simulink model "modle"  (R2023a)
settings: Solver=VariableStepAuto  StartTime=0.0  StopTime=10  RelTol=1e-3
model workspace (MAT data in the model file):
  a = 0.05
(part 1 of 2)
settings Model: Creator=shenwei  LastModifiedBy=shenwei

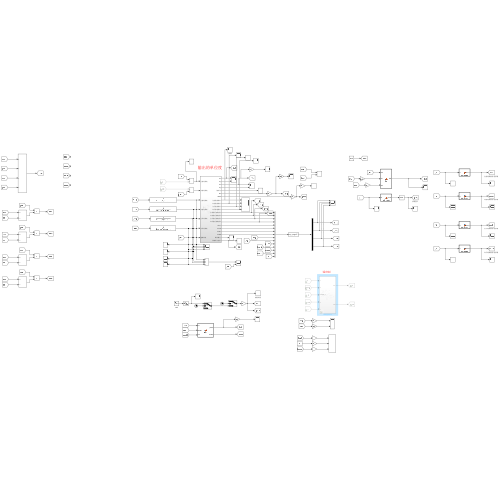
[thumbnail: Simulink's stored preview of the top-level diagram]
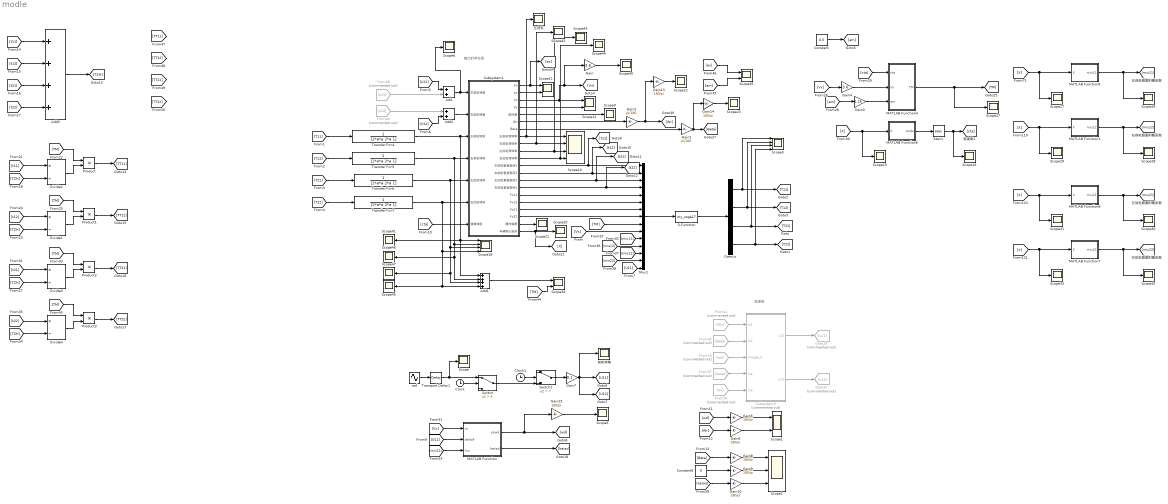
== system modle ==
  note: 输出的单位度
  note: 弧度制
  Add : Sum
  Add1 : Sum  Inputs=++++
  Add2 : Sum
  Add3 : Sum  Inputs=++++
  Atan1 : Trigonometry  Operator=atan
  Clock : Clock
  Clock1 : Clock
  Constant : Constant  Value=0.5
  Constant6 : Constant  Value=0
  Demux : Demux
  Divide{1..4} (4 alike) : Product  Inputs=*/
  From10 : From  Commented=on  GotoTag=wd
  From39 : From  Commented=on  GotoTag=u11
  From40 : From  Commented=on  GotoTag=u12
  From41 : From  Commented=on  GotoTag=Wr
  From42 : From  Commented=on  GotoTag=Beta
  From56 : From  Commented=on  GotoTag=Vx
  From57 : From  Commented=on  GotoTag=betad
  Gain : Gain  Gain=3.6
  Gain1 : Gain  Gain=pi/180
  Gain{5..6,8..10,13..15} (8 alike) : Gain  Gain=180/pi
  Gain2 : Gain  Gain=pi/180
  Gain3 : Gain  Gain=1.28
  Gain4 : Gain  Gain=3.6
  Gain7 : Gain  Gain=0.1
  Goto29 : Goto  Commented=on  GotoTag=u11
  Goto31 : Goto  Commented=on  GotoTag=u12
  MATLAB Function : MATLAB Function  TreatAsAtomicUnit=on
  MATLAB Function1 : MATLAB Function  TreatAsAtomicUnit=on
  MATLAB Function4 : MATLAB Function  TreatAsAtomicUnit=on
  MATLAB Function6 : MATLAB Function  TreatAsAtomicUnit=on
  MATLAB Function7 : MATLAB Function  TreatAsAtomicUnit=on
  MATLAB Function8 : MATLAB Function  TreatAsAtomicUnit=on
  MATLAB Function9 : MATLAB Function  TreatAsAtomicUnit=on
  Mux1 : Mux  Inputs=15
  Product{,1..3} (4 alike) : Product
  S-Function : S-Function  FunctionName=my_nsga17  SFunctionDeploymentMode=off  EnableBusSupport=off
  Scope{,5..6,9,16..17,19..23,26..33,40..47} (27 alike) : Scope
  Scope{1,11..12,34..35} (5 alike) : Scope  NumInputPorts=2
  Scope10 : Scope  NumInputPorts=4
  Scope18 : Scope  NumInputPorts=4
  Scope2 : Scope  NumInputPorts=3
  Scope3 : Scope  NumInputPorts=4
  Subsystem1 : Subsystem
  Subsystem3 : Subsystem  Commented=on
  Switch : Switch  Criteria=u2 > Threshold  Threshold=3  SaturateOnIntegerOverflow=off  InputSameDT=off
  Switch1 : Switch  Criteria=u2 > Threshold  Threshold=7  SaturateOnIntegerOverflow=off  InputSameDT=off
  Transfer Fcn{4..7} (4 alike) : TransferFcn  Denominator=[2*a*a 2*a 1]
  Transport Delay1 : TransportDelay  DelayTime=3
  rad : Sin  Amplitude=pi/4  Frequency=pi/2  SampleTime=0
  前轮转角 : Scope
  左前轮 : Scope
  wires:
  Subsystem1/12(左前轮垂直载荷1) -> [t11], Mux1/1
  Subsystem1/19(Fx22) -> Mux1/8
  Subsystem1/18(Fx21) -> Mux1/7
  Subsystem1/17(Fx12) -> Mux1/6
  Subsystem1/16(Fx11) -> Mux1/5
  Subsystem1/15(右后轮垂直载荷1) -> [t22], Mux1/4
  Subsystem1/14(左后轮垂直载荷1) -> Mux1/3, [t21]
  Subsystem1/13(右前轮垂直载荷1) -> Mux1/2, [t12]
  [TM] -> Mux1/9
  Demux/1 -> Scope3/1, [T11]
  Demux/2 -> Scope3/2, [T12]
  Demux/4 -> Scope3/4, [T22]
  Demux/3 -> Scope3/3, [T21]
  [Vx] -> Mux1/10
  Mux1/1 -> S-Function/1
  S-Function/1 -> Demux/1
  Subsystem1/11(右后轮滑转率) -> Scope44/1, Scope10/4
  Subsystem1/10(左后轮滑转率) -> Scope10/3, Scope43/1
  Subsystem1/9(右前轮滑转率) -> Scope42/1, Scope10/2
  Subsystem1/8(左前轮滑转率) -> Scope10/1, 左前轮/1
  Gain4/1 -> MATLAB Function4/2(Vx)
  MATLAB Function4/1(TM) -> Scope17/1, [TM]
  [cta] -> MATLAB Function4/1(cta)
  [am] -> Gain3/1
  MATLAB Function6/1(podu) -> Atan1/1
  [Vx] -> Gain4/1
  Atan1/1 -> Scope16/1, [cta]
  [cta] -> Subsystem1/7(道路坡度)
  Subsystem1/2(ay) -> Scope11/2
  Subsystem1/4(Vy) -> Scope12/2
  Subsystem1/3(Vx) -> Gain/1, [Vx], Scope12/1
  [X] -> Scope19/1, MATLAB Function6/1(X)
  Gain3/1 -> MATLAB Function4/3(am)
  Transfer Fcn4/1 -> Scope41/1, Scope18/1, Add1/1, Subsystem1/3(左前轮转矩)
  Transfer Fcn7/1 -> Scope45/1, Add1/4, Scope18/4, Subsystem1/6(右后轮转矩)
  Transfer Fcn6/1 -> Scope18/3, Scope47/1, Add1/3, Subsystem1/5(左后轮转矩)
  Transfer Fcn5/1 -> Scope18/2, Scope46/1, Add1/2, Subsystem1/4(右前轮转矩)
  Subsystem1/1(ax) -> [ax], Scope11/1
  MATLAB Function7/1(miu22) -> Scope32/1, [miu22]
  [X] -> Scope31/1, MATLAB Function8/1(X)
  [X] -> Scope33/1, MATLAB Function7/1(X)
  MATLAB Function8/1(miu21) -> Scope30/1, [miu21]
  MATLAB Function9/1(miu11) -> Scope26/1, [miu11]
  [X] -> Scope29/1, MATLAB Function1/1(X)
  [X] -> Scope27/1, MATLAB Function9/1(X)
  MATLAB Function1/1(miu12) -> Scope28/1, [miu12]
  Subsystem1/21(车辆质心坐标) -> Scope20/1, [X]
  [miu11] -> Mux1/11
  [miu12] -> Mux1/12
  [miu21] -> Mux1/13
  [miu22] -> Mux1/14
  Subsystem1/20(横向偏差) -> Scope21/1
  Subsystem1/7(Beta) -> Gain1/1
  Subsystem1/5(航向角) -> Scope9/1
  Subsystem1/6(Wr) -> Gain2/1
  From57/1 -> Subsystem3/4(In4)
  From42/1 -> Subsystem3/2(In2)
  From41/1 -> Subsystem3/1(In1)
  Add1/1 -> Scope34/1
  [TM] -> Scope34/2
  [ax] -> Scope35/1
  [am] -> Scope35/2
  Gain/1 -> Scope40/1
  Constant/1 -> [am]
  Clock1/1 -> Switch1/2
  Switch1/1 -> Gain7/1
  Switch/1 -> Switch1/3
  Transport Delay1/1 -> Switch/1, Scope/1
  Clock/1 -> Switch/2
  rad/1 -> Transport Delay1/1
  [U11] -> Add/1
  From39/1 -> Add/2
  [U12] -> Add2/2
  From40/1 -> Add2/1
  Add/1 -> Scope6/1, Subsystem1/1(左前轮转角)
  Add2/1 -> Subsystem1/2(右前轮转角)
  [U11] -> Mux1/15
  [wd] -> Gain5/1
  [Beta] -> Gain8/1
  Constant6/1 -> Gain9/1
  From10/1 -> Subsystem3/3(omega_d)
  [Wr] -> Gain6/1
  Subsystem3/1(u11) -> Goto29/1
  Subsystem3/2(u12) -> Goto31/1
  [t22] -> Add3/4
  [t11] -> Add3/1
  [t12] -> Add3/2
  [t21] -> Add3/3
  Add3/1 -> [TZH]
  [TZH] -> Divide2/2
  [t11] -> Divide2/1
  Divide2/1 -> Product/2
  [TM] -> Product/1
  Product/1 -> [TT11]
  Divide1/1 -> Product1/2
  [t12] -> Divide1/1
  [TZH] -> Divide1/2
  Product1/1 -> [TT12]
  [TM] -> Product1/1
  Divide3/1 -> Product2/2
  [t21] -> Divide3/1
  [TZH] -> Divide3/2
  Product2/1 -> [TT21]
  [TM] -> Product2/1
  Divide4/1 -> Product3/2
  [t22] -> Divide4/1
  [TZH] -> Divide4/2
  Product3/1 -> [TT22]
  [TM] -> Product3/1
  [Vx] -> MATLAB Function/1(vx)
  [miu11] -> MATLAB Function/3(mu)
  Gain7/1 -> [U12], 前轮转角/1, [U11]
  MATLAB Function/2(betad) -> [betad]
  Gain2/1 -> Gain13/1, [Wr]
  Gain1/1 -> Gain14/1, [Beta]
  Gain5/1 -> Scope1/1
  Gain9/1 -> Scope2/2
  Gain8/1 -> Scope2/1
  Gain6/1 -> Scope1/2
  [betad] -> Gain10/1
  Gain10/1 -> Scope2/3
  MATLAB Function/1(yawd) -> Gain15/1, [wd]
  [U11] -> MATLAB Function/2(deltaf)
  Gain13/1 -> Scope22/1
  Gain14/1 -> Scope23/1
  From56/1 -> Subsystem3/5(In3)
  Gain15/1 -> Scope5/1
  [T11] -> Transfer Fcn4/1
  [T12] -> Transfer Fcn5/1
  [T21] -> Transfer Fcn6/1
  [T22] -> Transfer Fcn7/1

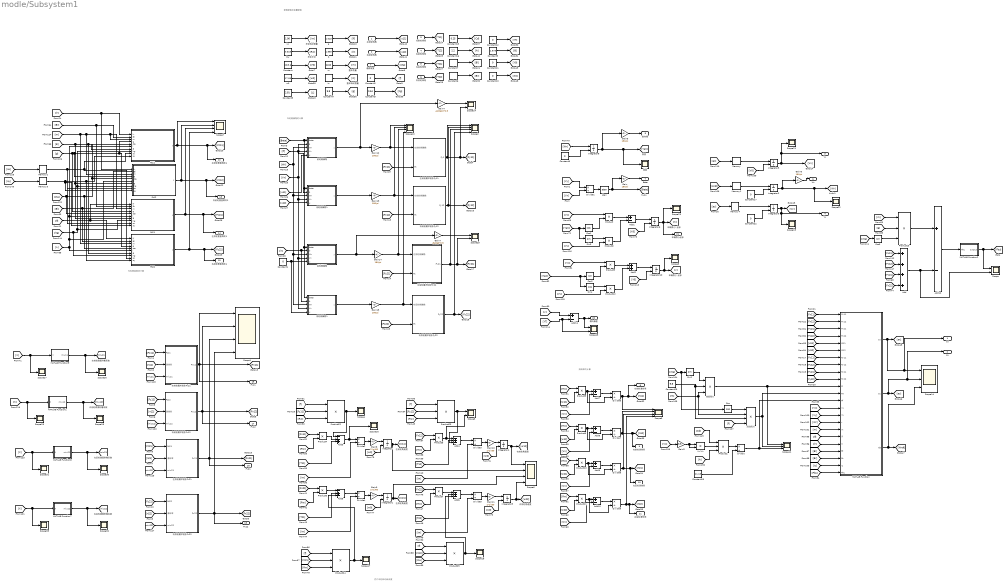
== system modle/Subsystem1 ==
  note: 滑转率的计算
  note: 四个车轮转动自由度
  note: 参数赋值及变量赋值
  note: 车轮侧偏角的计算
  note: 车轮垂直载荷计算
  左前轮转角 : Inport
  右前轮转角 : Inport  Port=2
  左前轮转矩 : Inport  Port=3
  右前轮转矩 : Inport  Port=4
  左后轮转矩 : Inport  Port=5
  右后轮转矩 : Inport  Port=6
  道路坡度 : Inport  Port=7
  Add : Sum  Inputs=++++
  Add{1,7..12} (7 alike) : Sum  Inputs=+-
  Add2 : Sum
  Add3 : Sum  Inputs=--+
  Add4 : Sum  Inputs=-+-
  Add5 : Sum  Inputs=-+-
  Add6 : Sum  Inputs=-+-
  Atan : Trigonometry  Operator=atan
  Constant : Constant  Value=20/3.6
  Constant{1..2,9..12,17,22} (8 alike) : Constant  Value=0
  Constant15 : Constant  Value=0.25
  Constant16 : Constant  Value=2.2
  Constant25 : Constant  Value=9.8
  Constant26 : Constant  Value=21.15
  Constant3 : Constant  Value=1.675
  Constant4 : Constant  Value=9.8
  Constant5 : Constant  Value=0.54
  Constant6 : Constant  Value=0.8375
  Constant7 : Constant  Value=0.8375
  Constant8 : Constant  Value=2.91
  Cos : Trigonometry  Operator=cos
  Cos1 : Trigonometry  Operator=cos
  Cos2 : Trigonometry
  Cos3 : Trigonometry
  Divide{1..9} (9 alike) : Product  Inputs=*/
  From150 : From
  Fz11 : MATLAB Function  TreatAsAtomicUnit=on
  Fz12 : MATLAB Function  TreatAsAtomicUnit=on
  Fz21 : MATLAB Function  TreatAsAtomicUnit=on
  Fz22 : MATLAB Function  TreatAsAtomicUnit=on
  Gain{,5..6,12..15} (7 alike) : Gain  Gain=180/pi
  Gain{8..11} (4 alike) : Gain  Gain=2*pi/60
  Gain3 : Gain  Gain=3.6
  Gain4 : Gain  Gain=-118610*0.5
  Gain7 : Gain  Gain=-94860*0.5
  Goto42 : Goto
  Integrator{,1..6,8..10} (10 alike) : Integrator  InitialConditionSource=external
  Iw : Constant  Value=1.06
  Iz : Constant  Value=1536.7
  MATLAB Function : MATLAB Function  TreatAsAtomicUnit=on
  MATLAB Function1 : MATLAB Function  TreatAsAtomicUnit=on
  MATLAB Function2 : MATLAB Function  TreatAsAtomicUnit=on
  MATLAB Function7 : MATLAB Function  TreatAsAtomicUnit=on
  MATLAB Function8 : MATLAB Function  TreatAsAtomicUnit=on
  MATLAB Function9 : MATLAB Function  TreatAsAtomicUnit=on
  Memory{,1..4} (5 alike) : Memory
  Product{,2..12} (12 alike) : Product
  Product{1,13,22..25} (6 alike) : Product  Inputs=3
  Rw : Constant  Value=0.325
  Scope{,5,15,24..25} (5 alike) : Scope  NumInputPorts=2
  Scope{1..2,6..7,9..10} (6 alike) : Scope  NumInputPorts=4
  Scope11 : Scope  NumInputPorts=3
  Scope14 : Scope  NumInputPorts=3
  Scope{4,8,16..19,21..23,26..33} (17 alike) : Scope
  Sin2 : Trigonometry
  Sin3 : Trigonometry
  Sin4 : Trigonometry  Operator=cos
  Vx*Vx : Product
  a : Constant  Value=1.015
  b : Constant  Value=1.895
  m : Constant  Value=1412
  w0 : Constant  Value=17.09
  前轮侧偏角 : MATLAB Function  TreatAsAtomicUnit=on
  前轮侧偏角1 : MATLAB Function  TreatAsAtomicUnit=on
  右前轮魔术轮胎Fx12 : Subsystem
  右前轮魔术轮胎Fy12 : Subsystem
  右后轮魔术轮胎Fx22 : Subsystem
  右后轮魔术轮胎Fy22 : Subsystem
  后轮侧偏角 : MATLAB Function  TreatAsAtomicUnit=on
  后轮侧偏角1 : MATLAB Function  TreatAsAtomicUnit=on
  坡度阻力 : Product  Inputs=3
  左前轮魔术轮胎Fx11 : Subsystem
  左前轮魔术轮胎Fy11 : Subsystem
  左后轮魔术轮胎Fx21 : Subsystem
  左后轮魔术轮胎Fy21 : Subsystem
  滚动阻力 : Product  Inputs=4
  空气阻力 : Product  Inputs=*/
  虎度 : Scope
  ax : Outport
  ay : Outport  Port=2
  Vx : Outport  Port=3
  Vy : Outport  Port=4
  航向角 : Outport  Port=5
  Wr : Outport  Port=6
  Beta : Outport  Port=7
  左前轮滑转率 : Outport  Port=8
  右前轮滑转率 : Outport  Port=9
  左后轮滑转率 : Outport  Port=10
  右后轮滑转率 : Outport  Port=11
  左前轮垂直载荷1 : Outport  Port=12
  右前轮垂直载荷1 : Outport  Port=13
  左后轮垂直载荷1 : Outport  Port=14
  右后轮垂直载荷1 : Outport  Port=15
  Fx11 : Outport  Port=16
  Fx12 : Outport  Port=17
  Fx21 : Outport  Port=18
  Fx22 : Outport  Port=19
  横向偏差 : Outport  Port=20
  车辆质心坐标 : Outport  Port=21
  wires:
  Product8/1 -> Divide6/2, Add7/1
  [Fz11] -> 左前轮魔术轮胎Fy11/2(Fz)
  右前轮魔术轮胎Fx12/1(Fx12) -> Fx12/1, Scope1/2, [Fx12]
  Add5/1 -> Divide4/1
  [Fz21] -> 左后轮魔术轮胎Fx21/1(Fz21)
  Product9/1 -> Divide7/2, Add8/1
  Iw/1 -> [Iw]
  [w0] -> Integrator4/2
  [Rw] -> Product9/1
  b/1 -> [lr]
  左前轮转矩/1 -> [T11]
  [Rw] -> Product4/2
  [Fz12] -> 右前轮魔术轮胎Fx12/1(Fz12)
  Add6/1 -> Divide5/1
  Divide5/1 -> Gain11/1
  [Rw] -> Product5/2
  [Fx12] -> Product5/1
  Product4/1 -> Add3/2
  Add7/1 -> Divide6/1
  [w12] -> Product9/2
  Iz/1 -> [Iz]
  右后轮魔术轮胎Fx22/1(Fx22) -> [Fx22], Fx22/1, Scope1/4
  [n12] -> 右前轮魔术轮胎Fx12/2(滑转率)
  Divide8/1 -> Scope9/3, 左后轮滑转率/1, [n21]
  Product11/1 -> Divide9/2, Add10/1
  Divide3/1 -> Gain10/1
  Product5/1 -> Scope5/2, Add4/1
  m/1 -> [m]
  [Fz11] -> 左前轮魔术轮胎Fx11/1(Fz11)
  [Fz22] -> 右后轮魔术轮胎Fy22/2(Fz)
  [w0] -> Integrator/2
  Constant/1 -> [V0]
  [Iw] -> Divide5/2
  Product7/1 -> Add6/1
  [Rw] -> Product7/2
  左后轮转矩/1 -> [T21]
  Product10/1 -> Divide8/2, Add9/1
  [Iw] -> Divide3/2
  Divide9/1 -> Scope9/4, 右后轮滑转率/1, [n22]
  Add4/1 -> Divide3/1
  [Fx22] -> Product7/1
  Integrator1/1 -> Scope6/3, [w21]
  Add9/1 -> Divide8/1
  [w11] -> Product8/2
  Add3/1 -> Scope16/1, Divide2/1
  [n11] -> 左前轮魔术轮胎Fx11/2(滑转率)
  [T22] -> Add6/2
  Gain15/1 -> 右后轮魔术轮胎Fy22/1(右后轮侧偏角), Scope10/4
  Gain14/1 -> Scope10/3, 左后轮魔术轮胎Fy21/1(左后轮侧偏角)
  [Vx] -> Add7/2
  [Rw] -> Product10/1
  [Vx] -> Add10/2
  Gain11/1 -> Integrator5/1
  Integrator4/1 -> [w12], Scope6/1
  [T12] -> Add4/2
  [w21] -> Product10/2
  右后轮转矩/1 -> [T22]
  Divide4/1 -> Gain9/1
  左前轮转角/1 -> [u11]
  Divide7/1 -> Scope9/2, 右前轮滑转率/1, [n12]
  [Rw] -> Product11/1
  Gain12/1 -> Scope10/1, 左前轮魔术轮胎Fy11/1(左前轮侧偏角)
  Gain9/1 -> Integrator1/1
  w0/1 -> [w0]
  [Fz21] -> 左后轮魔术轮胎Fy21/2(Fz)
  Product6/1 -> Add5/1
  [Vx] -> Add9/2
  Divide2/1 -> Gain8/1
  [Iw] -> Divide2/2
  Add8/1 -> Divide7/1
  [T11] -> Add3/3
  Gain13/1 -> Scope10/2, 右前轮魔术轮胎Fy12/1(右前轮侧偏角)
  a/1 -> [lf]
  [w0] -> Integrator1/2
  [w0] -> Integrator5/2
  [Vx] -> Add8/2
  Integrator/1 -> Scope6/2, [w11]
  Gain10/1 -> Integrator4/1
  Rw/1 -> [Rw]
  右前轮转矩/1 -> [T12]
  Divide6/1 -> Scope9/1, 左前轮滑转率/1, [n11]
  [Fx21] -> Product6/1
  Add10/1 -> Divide9/1
  Integrator5/1 -> Scope6/4, [w22]
  [Fx11] -> Product4/1
  [w22] -> Product11/2
  右前轮转角/1 -> [u12]
  [Iw] -> Divide4/2
  [Fz12] -> 右前轮魔术轮胎Fy12/2(Fz)
  [Rw] -> Product6/2
  [Rw] -> Product8/1
  [Fz21] -> 右后轮魔术轮胎Fx22/1(Fz22)
  Gain8/1 -> Integrator/1
  [T21] -> Add5/2
  [n21] -> 左后轮魔术轮胎Fx21/2(滑转率)
  [n22] -> 右后轮魔术轮胎Fx22/2(滑转率)
  道路坡度/1 -> [cta]
  [Wr] -> 前轮侧偏角1/3(Wr), 后轮侧偏角/3(Wr), 后轮侧偏角1/3(Wr), 前轮侧偏角/3(Wr)
  [lr] -> 后轮侧偏角/2(b), 后轮侧偏角1/2(b)
  [Vx] -> 前轮侧偏角1/4(Vx), 后轮侧偏角/4(Vx), 后轮侧偏角1/4(Vx), 前轮侧偏角/4(Vx)
  [u11] -> 前轮侧偏角/5(u)
  Constant1/1 -> 后轮侧偏角1/5(u), 后轮侧偏角/5(u)
  [Beta] -> 前轮侧偏角1/1(beta), 后轮侧偏角1/1(beta), 后轮侧偏角/1(beta), 前轮侧偏角/1(beta)
  [lf] -> 前轮侧偏角1/2(a), 前轮侧偏角/2(a)
  [u12] -> 前轮侧偏角1/5(u)
  [f] -> Product22/1
  [Fz11] -> Product22/2
  [Rw] -> Product22/3
  Constant2/1 -> [f]
  Product22/1 -> Scope4/1, Add3/1
  Product23/1 -> Add4/3, Scope5/1
  [Fz12] -> Product23/2
  [Rw] -> Product23/3
  [f] -> Product23/1
  Product24/1 -> Scope17/1, Add5/3
  [Fz21] -> Product24/2
  [Rw] -> Product24/3
  [f] -> Product24/1
  Product25/1 -> Add6/3, Scope18/1
  [Fz22] -> Product25/2
  [Rw] -> Product25/3
  [f] -> Product25/1
  [Vx] -> MATLAB Function/14(Vx)
  From150/1 -> Product1/3
  [V0] -> Integrator3/2
  坡度阻力/1 -> Scope11/1, MATLAB Function/11(Fi)
  Constant17/1 -> Integrator2/2
  [Vx] -> Gain3/1
  [Br] -> MATLAB Function/21(Br)
  [u11] -> MATLAB Function/5(O11)
  [m] -> 坡度阻力/3, 滚动阻力/2
  [Fx21] -> MATLAB Function/3(Fx21)
  [m] -> MATLAB Function/17(m)
  Constant26/1 -> 空气阻力/2
  MATLAB Function/2(ay) -> ay/1, Scope14/2, [ay]
  [Bl] -> MATLAB Function/20(Bl)
  [Iz] -> MATLAB Function/22(Iz)
  Cos/1 -> 滚动阻力/1
  Sin2/1 -> 坡度阻力/1
  MATLAB Function/1(ax) -> ax/1, Scope14/1, [ax]
  Gain3/1 -> Vx*Vx/2, Vx*Vx/1
  滚动阻力/1 -> Scope11/2, MATLAB Function/12(Fw)
  [Fy12] -> MATLAB Function/8(Fy12)
  Constant22/1 -> Integrator9/2
  [Fy21] -> MATLAB Function/9(Fy21)
  [lf] -> MATLAB Function/18(lf)
  [Fy22] -> MATLAB Function/10(Fy22)
  空气阻力/1 -> MATLAB Function/13(Ff), Scope11/3
  [Fy11] -> MATLAB Function/7(Fy11)
  Product1/1 -> 空气阻力/1
  Integrator9/1 -> Vy/1, Scope19/1, [Vy]
  [Fx22] -> MATLAB Function/4(Fx22)
  [Cd] -> Product1/1
  [Wr] -> MATLAB Function/16(r)
  Integrator3/1 -> Vx/1, Scope21/1, [Vx]
  Vx*Vx/1 -> Product1/2
  Integrator2/1 -> Gain6/1, Scope22/1, [Wr]
  [Fx11] -> MATLAB Function/1(Fx11)
  Constant25/1 -> 滚动阻力/3, 坡度阻力/2
  [lr] -> MATLAB Function/19(lr)
  [Fx12] -> MATLAB Function/2(Fx12)
  [Vy] -> MATLAB Function/15(Vy)
  [cta] -> Cos/1, Sin2/1
  [u12] -> MATLAB Function/6(O12)
  MATLAB Function/3(rdt) -> Scope14/3, [Wrdt]
  [f] -> 滚动阻力/4
  右前轮魔术轮胎Fy12/1(Fy12) -> Scope2/2, [Fy12]
  左前轮魔术轮胎Fy11/1(Fy1) -> Scope2/1, Scope24/2, [Fy11]
  Constant16/1 -> Goto42/1
  Constant7/1 -> [Bl]
  Constant6/1 -> [Br]
  Constant15/1 -> [Cd]
  右后轮魔术轮胎Fy22/1(Fy22) -> Scope2/4, [Fy22]
  Fz21/1(y) -> Scope7/3, 左后轮垂直载荷1/1, [Fz21]
  Fz12/1(y) -> 右前轮垂直载荷1/1, [Fz12], Scope7/2
  Memory3/1 -> Fz12/10(ay), Fz21/10(ay), Fz22/10(ay), Fz11/10(ay)
  [lf] -> Fz22/1(lf), Fz21/1(lf)
  [g] -> Fz22/4(g), Fz11/4(g), Fz12/4(g), Fz21/4(g)
  [lr] -> Fz11/1(lr), Fz12/1(lr)
  Fz11/1(y) -> 左前轮垂直载荷1/1, [Fz11], Scope7/1
  Memory2/1 -> Fz21/9(ax), Fz22/9(ax), Fz11/9(ax), Fz12/9(ax)
  [hg] -> Fz22/8(hg), Fz21/8(hg), Fz12/8(hg), Fz11/8(hg)
  [L] -> Fz22/6(l), Fz21/6(l), Fz11/6(l), Fz12/6(l)
  [Bl] -> Fz22/2(Bl), Fz12/2(Bl)
  [B] -> Fz21/7(B), Fz12/7(B), Fz22/7(B), Fz11/7(B)
  [Br] -> Fz21/2(Br), Fz11/2(Br)
  [cta] -> Fz21/5(cta), Fz22/5(cta), Fz12/5(cta), Fz11/5(cta)
  [m] -> Fz22/3(m), Fz21/3(m), Fz11/3(m), Fz12/3(m)
  Constant3/1 -> [B]
  Constant4/1 -> [g]
  Constant5/1 -> [hg]
  Constant8/1 -> [L]
  Fz22/1(y) -> Scope7/4, 右后轮垂直载荷1/1, [Fz22]
  [ax] -> Memory2/1
  [ay] -> Memory3/1
  Add11/1 -> Scope15/1, 横向偏差/1
  [Vy] -> Product12/2
  [Vx] -> Product3/1
  Product2/1 -> Add1/2
  Add1/1 -> Integrator6/1
  [YT] -> Scope15/2, Add11/2
  Product12/1 -> Add2/2
  Constant9/1 -> Integrator8/2
  Sin4/1 -> Product12/1
  [Wr] -> Integrator8/1
  Integrator10/1 -> Scope8/1, [y]
  Add2/1 -> Integrator10/1
  [X0] -> Integrator6/2
  Cos2/1 -> Product3/2
  [Vy] -> Product2/2
  [Vx] -> Product/1
  Sin3/1 -> Product2/1
  Product3/1 -> Add2/1
  Integrator6/1 -> 车辆质心坐标/1, Scope23/1, [X]
  Integrator8/1 -> 虎度/1, [Yaw], Gain5/1
  Cos1/1 -> Product/2
  [y] -> Add11/1
  Product/1 -> Add1/1
  [Y0] -> Integrator10/2
  Constant10/1 -> [X0]
  Constant11/1 -> [Y0]
  Constant12/1 -> [YT]
  Gain5/1 -> 航向角/1
  Gain6/1 -> Wr/1
  [Yaw] -> Sin3/1, Cos1/1
  [Yaw] -> Sin4/1, Cos2/1
  左前轮魔术轮胎Fx11/1(Fx11) -> [Fx11], Fx11/1, Scope1/1
  左后轮魔术轮胎Fx21/1(Fx21) -> Scope1/3, [Fx21], Fx21/1
  左后轮魔术轮胎Fy21/1(Fy21) -> Scope25/2, [Fy21], Scope2/3
  [miu11] -> 左前轮魔术轮胎Fx11/3(miu11)
  [miu12] -> 右前轮魔术轮胎Fx12/3(miu12)
  [miu21] -> 左后轮魔术轮胎Fx21/3(miu21)
  [miu22] -> 右后轮魔术轮胎Fx22/3(miu22)
  后轮侧偏角/1(y) -> Gain7/1, Gain14/1
  前轮侧偏角1/1(y) -> Gain13/1
  前轮侧偏角/1(y) -> Gain4/1, Gain12/1
  后轮侧偏角1/1(y) -> Gain15/1
  Gain4/1 -> Scope24/1
  Gain7/1 -> Scope25/1
  Divide1/1 -> Atan/1
  Atan/1 -> Gain/1, [Beta]
  [Vx] -> Divide1/2
  [Vy] -> Divide1/1
  [ax] -> Memory/1
  [ay] -> Memory4/1
  [Wrdt] -> Memory1/1
  Memory/1 -> Integrator3/1
  Memory4/1 -> Integrator9/1
  Memory1/1 -> Integrator2/1
  [X] -> Scope31/1, MATLAB Function8/1(X)
  MATLAB Function9/1(miu11) -> Scope26/1, [miu11]
  [X] -> Scope33/1, MATLAB Function7/1(X)
  [X] -> Scope27/1, MATLAB Function9/1(X)
  [X] -> Scope29/1, MATLAB Function1/1(X)
  MATLAB Function8/1(miu21) -> Scope30/1, [miu21]
  MATLAB Function1/1(miu12) -> Scope28/1, [miu12]
  MATLAB Function7/1(miu22) -> Scope32/1, [miu22]
  [m] -> Product13/1
  Cos3/1 -> Product13/3
  [cta] -> Cos3/1
  [Fx22] -> Add/4
  [Fx11] -> Add/1
  Add/1 -> Scope/2, Add12/2
  [Fx21] -> Add/3
  [Fx12] -> Add/2
  MATLAB Function2/1(output) -> Scope/1, [Fbu]
  Product13/1 -> Add12/1
  [g] -> Product13/2
  Add12/1 -> MATLAB Function2/1(Fbu)
  [Fbu] -> MATLAB Function/23(Fbu)
  Gain/1 -> Beta/1

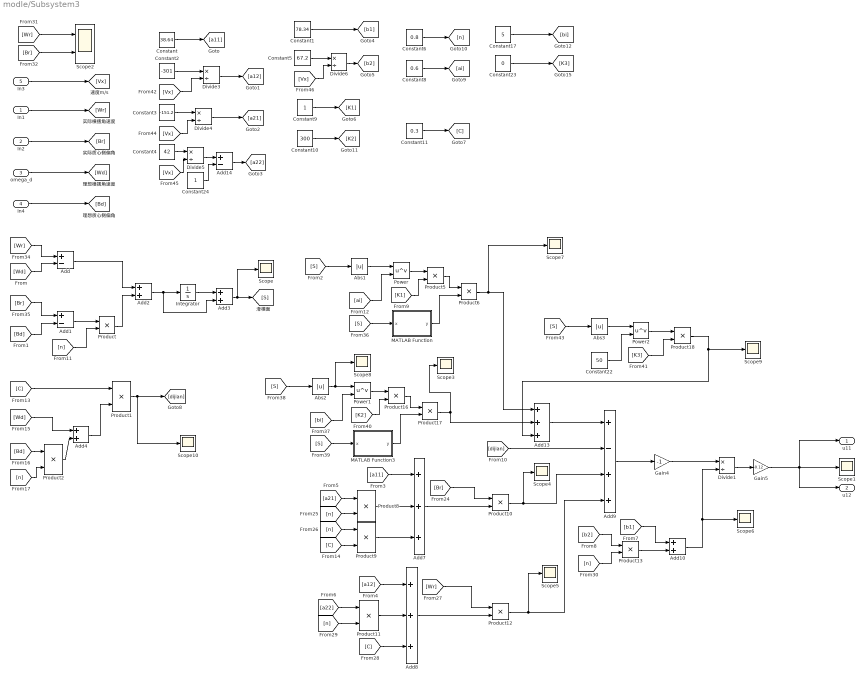
== system modle/Subsystem3 ==
  In1 : Inport
  In2 : Inport  Port=2
  omega_d : Inport  Port=3
  In4 : Inport  Port=4
  In3 : Inport  Port=5
  Abs1 : Abs  SaturateOnIntegerOverflow=off
  Abs2 : Abs  SaturateOnIntegerOverflow=off
  Abs3 : Abs  SaturateOnIntegerOverflow=off
  Add : Sum  Inputs=+-
  Add1 : Sum  Inputs=+-
  Add{2..4,10} (4 alike) : Sum
  Add13 : Sum  Inputs=+++
  Add14 : Sum  Inputs=+-
  Add7 : Sum  Inputs=+++
  Add8 : Sum  Inputs=+++
  Add9 : Sum  Inputs=+-++
  Constant : Constant  Value=38.64
  Constant1 : Constant  Value=78.34
  Constant10 : Constant  Value=300
  Constant11 : Constant  Value=0.3
  Constant17 : Constant  Value=5
  Constant2 : Constant  Value=-301
  Constant22 : Constant  Value=50
  Constant23 : Constant  Value=0
  Constant24 : Constant
  Constant3 : Constant  Value=-151.2
  Constant4 : Constant  Value=42
  Constant5 : Constant  Value=67.2
  Constant6 : Constant  Value=0.8
  Constant8 : Constant  Value=0.6
  Constant9 : Constant
  Divide{1,3..6} (5 alike) : Product  Inputs=*/
  Gain4 : Gain  Gain=-1
  Gain5 : Gain  Gain=-0.12
  Integrator : Integrator
  MATLAB Function : MATLAB Function  TreatAsAtomicUnit=on
  MATLAB Function3 : MATLAB Function  TreatAsAtomicUnit=on
  Power : Math  Operator=pow
  Power1 : Math  Operator=pow
  Power2 : Math  Operator=pow
  Product{,1..2,5..6,8..13,16..18} (14 alike) : Product
  Scope{,1,3..10} (10 alike) : Scope
  Scope2 : Scope  NumInputPorts=2
  u11 : Outport
  u12 : Outport  Port=2
  wires:
  [Wr] -> Add/1
  [Wd] -> Add/2
  [Br] -> Add1/1
  [Bd] -> Add1/2
  Add1/1 -> Product/1
  [n] -> Product/2
  Add/1 -> Add2/1
  Product/1 -> Add2/2
  Add2/1 -> Add3/2, Integrator/1
  Integrator/1 -> Add3/1
  In1/1 -> [Wr]
  In4/1 -> [Bd]
  In2/1 -> [Br]
  Constant/1 -> [a11]
  Constant1/1 -> [b1]
  Constant9/1 -> [K1]
  Constant10/1 -> [K2]
  Constant6/1 -> [n]
  Constant8/1 -> [ai]
  Constant11/1 -> [C]
  [S] -> Abs1/1
  [K1] -> Product5/2
  Abs1/1 -> Power/1
  [ai] -> Power/2
  Power/1 -> Product5/1
  Product5/1 -> Product6/1
  [a11] -> Add7/1
  [a21] -> Product8/1
  [n] -> Product8/2
  Product8/1 -> Add7/2
  [n] -> Product9/1
  [C] -> Product9/2
  Product9/1 -> Add7/3
  Add7/1 -> Product10/2
  [Br] -> Product10/1
  [a12] -> Add8/1
  [C] -> Add8/3
  Product11/1 -> Add8/2
  Add8/1 -> Product12/2
  [Wr] -> Product12/1
  [a22] -> Product11/1
  [n] -> Product11/2
  Product10/1 -> Scope4/1, Add9/3
  Product12/1 -> Scope5/1, Add9/4
  Add9/1 -> Gain4/1
  [b2] -> Product13/1
  [n] -> Product13/2
  Product13/1 -> Add10/2
  [b1] -> Add10/1
  Gain4/1 -> Divide1/1
  Add10/1 -> Scope6/1, Divide1/2
  Divide1/1 -> Gain5/1
  Gain5/1 -> u12/1, Scope1/1, u11/1
  [Wr] -> Scope2/1
  [Br] -> Scope2/2
  [dijian] -> Add9/2
  Add3/1 -> Scope/1, [S]
  [S] -> MATLAB Function/1(x)
  MATLAB Function/1(y) -> Product6/2
  MATLAB Function3/1(y) -> Product17/2
  Abs2/1 -> Scope8/1, Power1/1
  Power1/1 -> Product16/1
  [S] -> Abs2/1
  [K2] -> Product16/2
  Product16/1 -> Product17/1
  [bi] -> Power1/2
  [S] -> MATLAB Function3/1(x)
  Constant17/1 -> [bi]
  Constant23/1 -> [K3]
  Abs3/1 -> Power2/1
  [S] -> Abs3/1
  Constant22/1 -> Power2/2
  Power2/1 -> Product18/1
  [K3] -> Product18/2
  Add13/1 -> Add9/1
  Product17/1 -> Scope3/1, Add13/2
  Product6/1 -> Scope7/1, Add13/1
  Product18/1 -> Add13/3, Scope9/1
  omega_d/1 -> [Wd]
  Constant2/1 -> Divide3/1
  [Vx] -> Divide3/2
  In3/1 -> [Vx]
  Divide3/1 -> [a12]
  Constant3/1 -> Divide4/1
  Divide4/1 -> [a21]
  [Vx] -> Divide4/2
  [Vx] -> Divide5/2
  Constant4/1 -> Divide5/1
  Divide5/1 -> Add14/1
  Add14/1 -> [a22]
  Constant24/1 -> Add14/2
  Constant5/1 -> Divide6/1
  [Vx] -> Divide6/2
  Divide6/1 -> [b2]
  [C] -> Product1/1
  [Wd] -> Add4/1
  [Bd] -> Product2/1
  Product2/1 -> Add4/2
  [n] -> Product2/2
  Add4/1 -> Product1/2
  Product1/1 -> Scope10/1, [dijian]

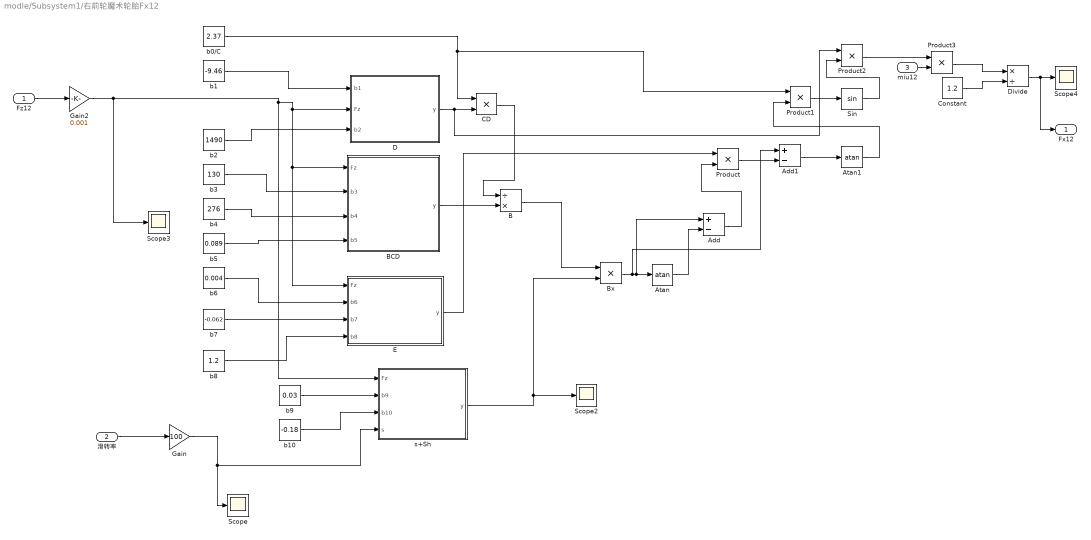
== system modle/Subsystem1/右前轮魔术轮胎Fx12 ==
  Fz12 : Inport
  滑转率 : Inport  Port=2
  miu12 : Inport  Port=3
  Add : Sum  Inputs=+-
  Add1 : Sum  Inputs=+-
  Atan : Trigonometry  Operator=atan
  Atan1 : Trigonometry  Operator=atan
  B : Product  Inputs=/*
  BCD : MATLAB Function  TreatAsAtomicUnit=on
  Bx : Product
  CD : Product
  Constant : Constant  Value=1.2  SampleTime=-1
  D : MATLAB Function  TreatAsAtomicUnit=on
  Divide : Product  Inputs=*/
  E : MATLAB Function  TreatAsAtomicUnit=on
  Gain : Gain  Gain=100
  Gain2 : Gain  Gain=0.001
  Product{,1..3} (4 alike) : Product
  Scope{,2..4} (4 alike) : Scope
  Sin : Trigonometry
  b0/C : Constant  Value=2.37
  b1 : Constant  Value=-9.46
  b10 : Constant  Value=-0.18
  b2 : Constant  Value=1490
  b3 : Constant  Value=130
  b4 : Constant  Value=276
  b5 : Constant  Value=0.089
  b6 : Constant  Value=0.004
  b7 : Constant  Value=-0.062
  b8 : Constant  Value=1.2
  b9 : Constant  Value=0.03
  s+Sh : MATLAB Function  TreatAsAtomicUnit=on
  Fx12 : Outport
  wires:
  Gain2/1 -> Scope3/1, s+Sh/1(Fz), E/1(Fz), BCD/1(Fz), D/2(Fz)
  b4/1 -> BCD/3(b4)
  Gain/1 -> s+Sh/4(s), Scope/1
  Product1/1 -> Sin/1
  滑转率/1 -> Gain/1
  b5/1 -> BCD/4(b5)
  Atan1/1 -> Product1/2
  Product/1 -> Add1/2
  D/1(y) -> Product2/1, CD/2
  b8/1 -> E/4(b8)
  Fz12/1 -> Gain2/1
  BCD/1(y) -> B/2
  B/1 -> Bx/1
  Add/1 -> Product/2
  b9/1 -> s+Sh/2(b9)
  Add1/1 -> Atan1/1
  b6/1 -> E/2(b6)
  b1/1 -> D/1(b1)
  Sin/1 -> Product2/2
  CD/1 -> B/1
  E/1(y) -> Product/1
  s+Sh/1(y) -> Scope2/1, Bx/2
  b10/1 -> s+Sh/3(b10)
  b2/1 -> D/3(b2)
  b7/1 -> E/3(b7)
  b3/1 -> BCD/2(b3)
  b0/C/1 -> Product1/1, CD/1
  Atan/1 -> Add/2
  Bx/1 -> Add1/1, Add/1, Atan/1
  Divide/1 -> Fx12/1, Scope4/1
  miu12/1 -> Product3/2
  Constant/1 -> Divide/2
  Product3/1 -> Divide/1
  Product2/1 -> Product3/1

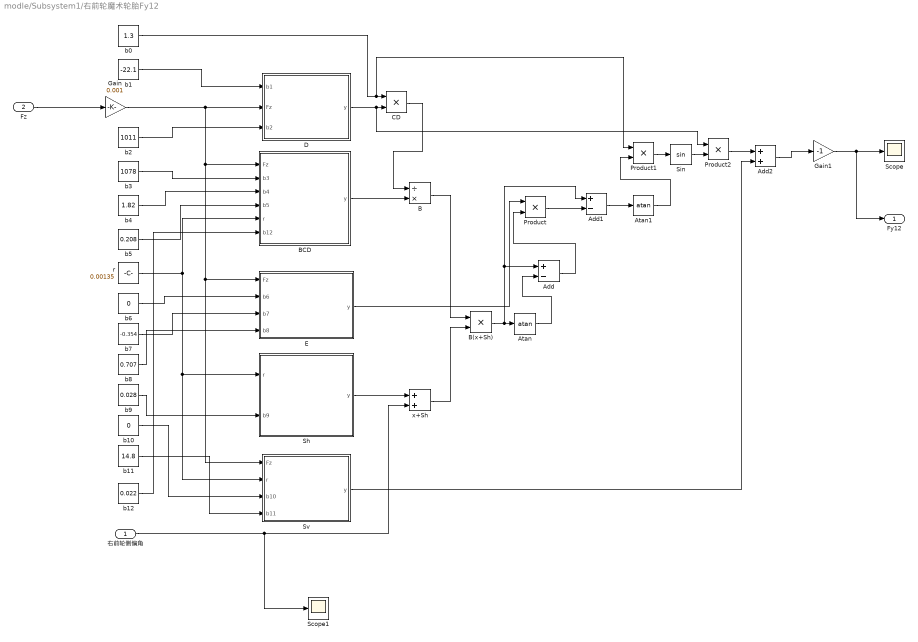
== system modle/Subsystem1/右前轮魔术轮胎Fy12 ==
  右前轮侧偏角 : Inport
  Fz : Inport  Port=2
  Add : Sum  Inputs=+-
  Add1 : Sum  Inputs=+-
  Add2 : Sum
  Atan : Trigonometry  Operator=atan
  Atan1 : Trigonometry  Operator=atan
  B : Product  Inputs=/*
  B(x+Sh) : Product
  BCD : MATLAB Function  TreatAsAtomicUnit=on
  CD : Product
  D : MATLAB Function  TreatAsAtomicUnit=on
  E : MATLAB Function  TreatAsAtomicUnit=on
  Gain : Gain  Gain=0.001
  Gain1 : Gain  Gain=-1
  Product : Product
  Product1 : Product
  Product2 : Product
  Scope : Scope
  Scope1 : Scope
  Sh : MATLAB Function  TreatAsAtomicUnit=on
  Sin : Trigonometry
  Sv : MATLAB Function  TreatAsAtomicUnit=on
  b0 : Constant  Value=1.3
  b1 : Constant  Value=-22.1
  b10 : Constant  Value=0
  b11 : Constant  Value=14.8
  b12 : Constant  Value=0.022
  b2 : Constant  Value=1011
  b3 : Constant  Value=1078
  b4 : Constant  Value=1.82
  b5 : Constant  Value=0.208
  b6 : Constant  Value=0
  b7 : Constant  Value=-0.354
  b8 : Constant  Value=0.707
  b9 : Constant  Value=0.028
  r : Constant  Value=0.00135
  x+Sh : Sum
  Fy12 : Outport
  wires:
  Gain1/1 -> Fy12/1, Scope/1
  b9/1 -> Sh/2(b9)
  右前轮侧偏角/1 -> Scope1/1, x+Sh/2
  r/1 -> Sv/2(r), Sh/1(r), BCD/5(r)
  Fz/1 -> Gain/1
  Atan/1 -> Add/2
  b0/1 -> Product1/1, CD/1
  b12/1 -> BCD/6(b12)
  b8/1 -> E/4(b8)
  b11/1 -> Sv/4(b11)
  Sin/1 -> Product2/2
  b4/1 -> BCD/3(b4)
  Add/1 -> Product/2
  B(x+Sh)/1 -> Add/1, Add1/1, Atan/1
  Sh/1(y) -> x+Sh/1
  D/1(y) -> Product2/1, CD/2
  B/1 -> B(x+Sh)/1
  Atan1/1 -> Product1/2
  b7/1 -> E/3(b7)
  CD/1 -> B/1
  b6/1 -> E/2(b6)
  BCD/1(y) -> B/2
  x+Sh/1 -> B(x+Sh)/2
  Product1/1 -> Sin/1
  E/1(y) -> Product/1
  Product/1 -> Add1/2
  b5/1 -> BCD/4(b5)
  Add1/1 -> Atan1/1
  b3/1 -> BCD/2(b3)
  b2/1 -> D/3(b2)
  b1/1 -> D/1(b1)
  b10/1 -> Sv/3(b10)
  Product2/1 -> Add2/1
  Sv/1(y) -> Add2/2
  Add2/1 -> Gain1/1
  Gain/1 -> Sv/1(Fz), E/1(Fz), BCD/1(Fz), D/2(Fz)

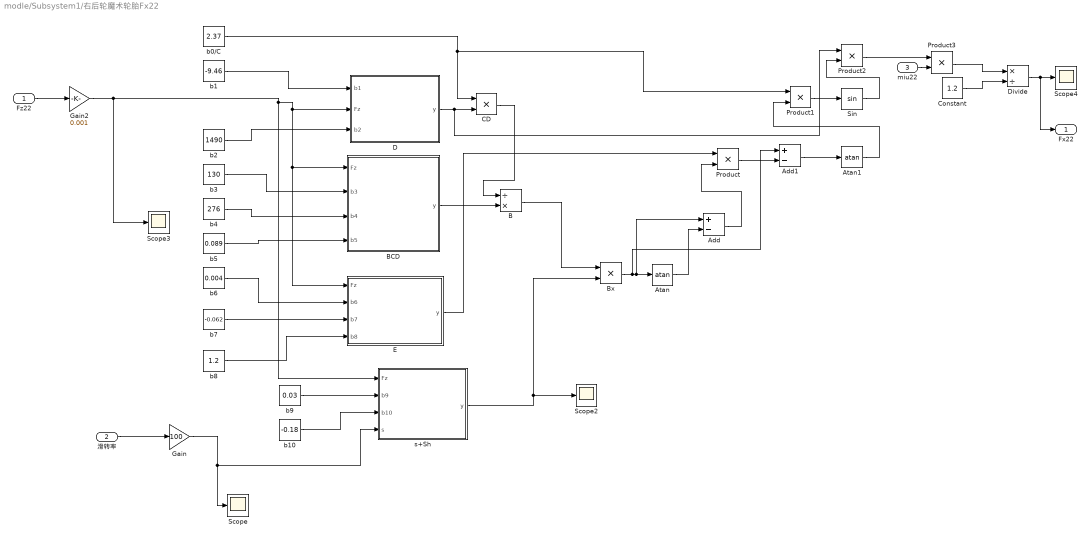
== system modle/Subsystem1/右后轮魔术轮胎Fx22 ==
  Fz22 : Inport
  滑转率 : Inport  Port=2
  miu22 : Inport  Port=3
  Add : Sum  Inputs=+-
  Add1 : Sum  Inputs=+-
  Atan : Trigonometry  Operator=atan
  Atan1 : Trigonometry  Operator=atan
  B : Product  Inputs=/*
  BCD : MATLAB Function  TreatAsAtomicUnit=on
  Bx : Product
  CD : Product
  Constant : Constant  Value=1.2  SampleTime=-1
  D : MATLAB Function  TreatAsAtomicUnit=on
  Divide : Product  Inputs=*/
  E : MATLAB Function  TreatAsAtomicUnit=on
  Gain : Gain  Gain=100
  Gain2 : Gain  Gain=0.001
  Product{,1..3} (4 alike) : Product
  Scope{,2..4} (4 alike) : Scope
  Sin : Trigonometry
  b0/C : Constant  Value=2.37
  b1 : Constant  Value=-9.46
  b10 : Constant  Value=-0.18
  b2 : Constant  Value=1490
  b3 : Constant  Value=130
  b4 : Constant  Value=276
  b5 : Constant  Value=0.089
  b6 : Constant  Value=0.004
  b7 : Constant  Value=-0.062
  b8 : Constant  Value=1.2
  b9 : Constant  Value=0.03
  s+Sh : MATLAB Function  TreatAsAtomicUnit=on
  Fx22 : Outport
  wires:
  Gain2/1 -> Scope3/1, s+Sh/1(Fz), E/1(Fz), BCD/1(Fz), D/2(Fz)
  b4/1 -> BCD/3(b4)
  Gain/1 -> s+Sh/4(s), Scope/1
  Product1/1 -> Sin/1
  滑转率/1 -> Gain/1
  b5/1 -> BCD/4(b5)
  Atan1/1 -> Product1/2
  Product/1 -> Add1/2
  D/1(y) -> Product2/1, CD/2
  b8/1 -> E/4(b8)
  Fz22/1 -> Gain2/1
  BCD/1(y) -> B/2
  B/1 -> Bx/1
  Add/1 -> Product/2
  b9/1 -> s+Sh/2(b9)
  Add1/1 -> Atan1/1
  b6/1 -> E/2(b6)
  b1/1 -> D/1(b1)
  Sin/1 -> Product2/2
  CD/1 -> B/1
  E/1(y) -> Product/1
  s+Sh/1(y) -> Scope2/1, Bx/2
  b10/1 -> s+Sh/3(b10)
  b2/1 -> D/3(b2)
  b7/1 -> E/3(b7)
  b3/1 -> BCD/2(b3)
  b0/C/1 -> Product1/1, CD/1
  Atan/1 -> Add/2
  Bx/1 -> Add1/1, Add/1, Atan/1
  Product3/1 -> Divide/1
  Divide/1 -> Fx22/1, Scope4/1
  miu22/1 -> Product3/2
  Product2/1 -> Product3/1
  Constant/1 -> Divide/2

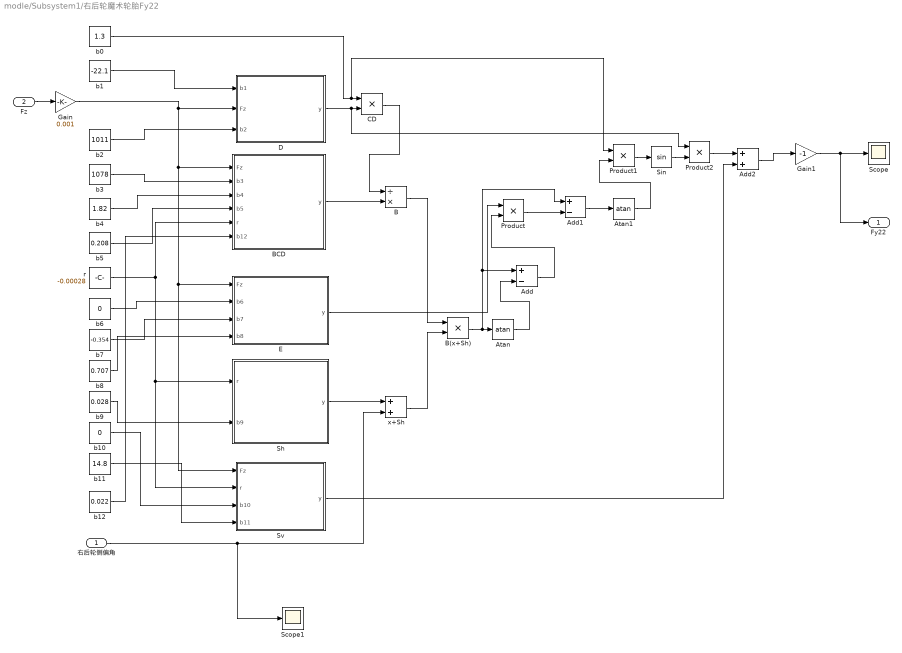
== system modle/Subsystem1/右后轮魔术轮胎Fy22 ==
  右后轮侧偏角 : Inport
  Fz : Inport  Port=2
  Add : Sum  Inputs=+-
  Add1 : Sum  Inputs=+-
  Add2 : Sum
  Atan : Trigonometry  Operator=atan
  Atan1 : Trigonometry  Operator=atan
  B : Product  Inputs=/*
  B(x+Sh) : Product
  BCD : MATLAB Function  TreatAsAtomicUnit=on
  CD : Product
  D : MATLAB Function  TreatAsAtomicUnit=on
  E : MATLAB Function  TreatAsAtomicUnit=on
  Gain : Gain  Gain=0.001
  Gain1 : Gain  Gain=-1
  Product : Product
  Product1 : Product
  Product2 : Product
  Scope : Scope
  Scope1 : Scope
  Sh : MATLAB Function  TreatAsAtomicUnit=on
  Sin : Trigonometry
  Sv : MATLAB Function  TreatAsAtomicUnit=on
  b0 : Constant  Value=1.3
  b1 : Constant  Value=-22.1
  b10 : Constant  Value=0
  b11 : Constant  Value=14.8
  b12 : Constant  Value=0.022
  b2 : Constant  Value=1011
  b3 : Constant  Value=1078
  b4 : Constant  Value=1.82
  b5 : Constant  Value=0.208
  b6 : Constant  Value=0
  b7 : Constant  Value=-0.354
  b8 : Constant  Value=0.707
  b9 : Constant  Value=0.028
  r : Constant  Value=-0.00028
  x+Sh : Sum
  Fy22 : Outport
  wires:
  Gain1/1 -> Fy22/1, Scope/1
  b9/1 -> Sh/2(b9)
  右后轮侧偏角/1 -> Scope1/1, x+Sh/2
  r/1 -> Sv/2(r), Sh/1(r), BCD/5(r)
  Fz/1 -> Gain/1
  Atan/1 -> Add/2
  b0/1 -> Product1/1, CD/1
  b12/1 -> BCD/6(b12)
  b8/1 -> E/4(b8)
  b11/1 -> Sv/4(b11)
  Sin/1 -> Product2/2
  b4/1 -> BCD/3(b4)
  Add/1 -> Product/2
  B(x+Sh)/1 -> Add/1, Add1/1, Atan/1
  Sh/1(y) -> x+Sh/1
  D/1(y) -> Product2/1, CD/2
  B/1 -> B(x+Sh)/1
  Atan1/1 -> Product1/2
  b7/1 -> E/3(b7)
  CD/1 -> B/1
  b6/1 -> E/2(b6)
  BCD/1(y) -> B/2
  x+Sh/1 -> B(x+Sh)/2
  Product1/1 -> Sin/1
  E/1(y) -> Product/1
  Product/1 -> Add1/2
  b5/1 -> BCD/4(b5)
  Add1/1 -> Atan1/1
  b3/1 -> BCD/2(b3)
  b2/1 -> D/3(b2)
  b1/1 -> D/1(b1)
  b10/1 -> Sv/3(b10)
  Product2/1 -> Add2/1
  Sv/1(y) -> Add2/2
  Add2/1 -> Gain1/1
  Gain/1 -> Sv/1(Fz), E/1(Fz), BCD/1(Fz), D/2(Fz)

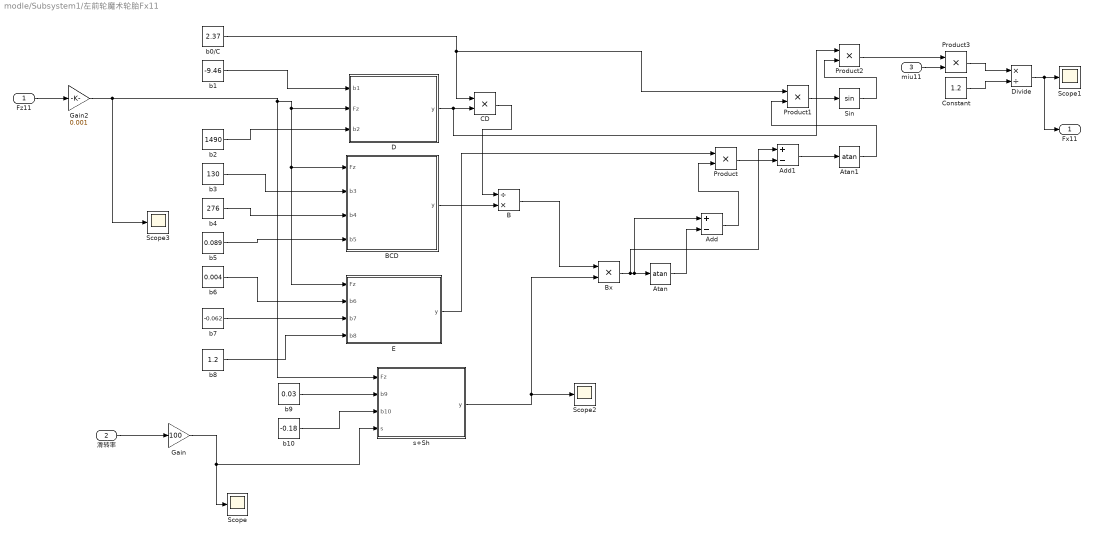
== system modle/Subsystem1/左前轮魔术轮胎Fx11 ==
  Fz11 : Inport
  滑转率 : Inport  Port=2
  miu11 : Inport  Port=3
  Add : Sum  Inputs=+-
  Add1 : Sum  Inputs=+-
  Atan : Trigonometry  Operator=atan
  Atan1 : Trigonometry  Operator=atan
  B : Product  Inputs=/*
  BCD : MATLAB Function  TreatAsAtomicUnit=on
  Bx : Product
  CD : Product
  Constant : Constant  Value=1.2  SampleTime=-1
  D : MATLAB Function  TreatAsAtomicUnit=on
  Divide : Product  Inputs=*/
  E : MATLAB Function  TreatAsAtomicUnit=on
  Gain : Gain  Gain=100
  Gain2 : Gain  Gain=0.001
  Product{,1..3} (4 alike) : Product
  Scope{,1..3} (4 alike) : Scope
  Sin : Trigonometry
  b0/C : Constant  Value=2.37
  b1 : Constant  Value=-9.46
  b10 : Constant  Value=-0.18
  b2 : Constant  Value=1490
  b3 : Constant  Value=130
  b4 : Constant  Value=276
  b5 : Constant  Value=0.089
  b6 : Constant  Value=0.004
  b7 : Constant  Value=-0.062
  b8 : Constant  Value=1.2
  b9 : Constant  Value=0.03
  s+Sh : MATLAB Function  TreatAsAtomicUnit=on
  Fx11 : Outport
  wires:
  Gain2/1 -> Scope3/1, s+Sh/1(Fz), E/1(Fz), BCD/1(Fz), D/2(Fz)
  b4/1 -> BCD/3(b4)
  Gain/1 -> s+Sh/4(s), Scope/1
  Product2/1 -> Product3/1
  Product1/1 -> Sin/1
  滑转率/1 -> Gain/1
  b5/1 -> BCD/4(b5)
  Atan1/1 -> Product1/2
  Product/1 -> Add1/2
  D/1(y) -> Product2/1, CD/2
  b8/1 -> E/4(b8)
  Fz11/1 -> Gain2/1
  BCD/1(y) -> B/2
  B/1 -> Bx/1
  Add/1 -> Product/2
  b9/1 -> s+Sh/2(b9)
  Add1/1 -> Atan1/1
  b6/1 -> E/2(b6)
  b1/1 -> D/1(b1)
  Sin/1 -> Product2/2
  E/1(y) -> Product/1
  s+Sh/1(y) -> Scope2/1, Bx/2
  b10/1 -> s+Sh/3(b10)
  b2/1 -> D/3(b2)
  b7/1 -> E/3(b7)
  b3/1 -> BCD/2(b3)
  b0/C/1 -> Product1/1, CD/1
  Atan/1 -> Add/2
  Bx/1 -> Add1/1, Add/1, Atan/1
  CD/1 -> B/1
  miu11/1 -> Product3/2
  Product3/1 -> Divide/1
  Constant/1 -> Divide/2
  Divide/1 -> Fx11/1, Scope1/1

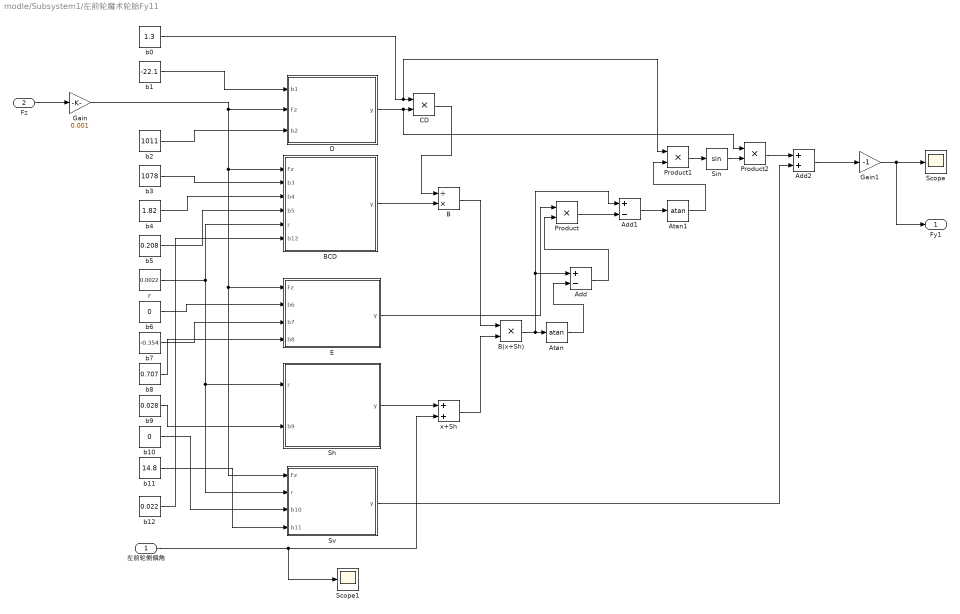
== system modle/Subsystem1/左前轮魔术轮胎Fy11 ==
  左前轮侧偏角 : Inport
  Fz : Inport  Port=2
  Add : Sum  Inputs=+-
  Add1 : Sum  Inputs=+-
  Add2 : Sum
  Atan : Trigonometry  Operator=atan
  Atan1 : Trigonometry  Operator=atan
  B : Product  Inputs=/*
  B(x+Sh) : Product
  BCD : MATLAB Function  TreatAsAtomicUnit=on
  CD : Product
  D : MATLAB Function  TreatAsAtomicUnit=on
  E : MATLAB Function  TreatAsAtomicUnit=on
  Gain : Gain  Gain=0.001
  Gain1 : Gain  Gain=-1
  Product : Product
  Product1 : Product
  Product2 : Product
  Scope : Scope
  Scope1 : Scope
  Sh : MATLAB Function  TreatAsAtomicUnit=on
  Sin : Trigonometry
  Sv : MATLAB Function  TreatAsAtomicUnit=on
  b0 : Constant  Value=1.3
  b1 : Constant  Value=-22.1
  b10 : Constant  Value=0
  b11 : Constant  Value=14.8
  b12 : Constant  Value=0.022
  b2 : Constant  Value=1011
  b3 : Constant  Value=1078
  b4 : Constant  Value=1.82
  b5 : Constant  Value=0.208
  b6 : Constant  Value=0
  b7 : Constant  Value=-0.354
  b8 : Constant  Value=0.707
  b9 : Constant  Value=0.028
  r : Constant  Value=0.0022
  x+Sh : Sum
  Fy1 : Outport
  wires:
  Gain1/1 -> Fy1/1, Scope/1
  b9/1 -> Sh/2(b9)
  左前轮侧偏角/1 -> Scope1/1, x+Sh/2
  r/1 -> Sv/2(r), Sh/1(r), BCD/5(r)
  Fz/1 -> Gain/1
  Atan/1 -> Add/2
  b0/1 -> Product1/1, CD/1
  b12/1 -> BCD/6(b12)
  b8/1 -> E/4(b8)
  b11/1 -> Sv/4(b11)
  Sin/1 -> Product2/2
  b4/1 -> BCD/3(b4)
  Add/1 -> Product/2
  B(x+Sh)/1 -> Add/1, Add1/1, Atan/1
  Sh/1(y) -> x+Sh/1
  D/1(y) -> Product2/1, CD/2
  B/1 -> B(x+Sh)/1
  Atan1/1 -> Product1/2
  b7/1 -> E/3(b7)
  CD/1 -> B/1
  b6/1 -> E/2(b6)
  BCD/1(y) -> B/2
  x+Sh/1 -> B(x+Sh)/2
  Product1/1 -> Sin/1
  E/1(y) -> Product/1
  Product/1 -> Add1/2
  b5/1 -> BCD/4(b5)
  Add1/1 -> Atan1/1
  b3/1 -> BCD/2(b3)
  b2/1 -> D/3(b2)
  b1/1 -> D/1(b1)
  b10/1 -> Sv/3(b10)
  Product2/1 -> Add2/1
  Sv/1(y) -> Add2/2
  Add2/1 -> Gain1/1
  Gain/1 -> Sv/1(Fz), E/1(Fz), BCD/1(Fz), D/2(Fz)

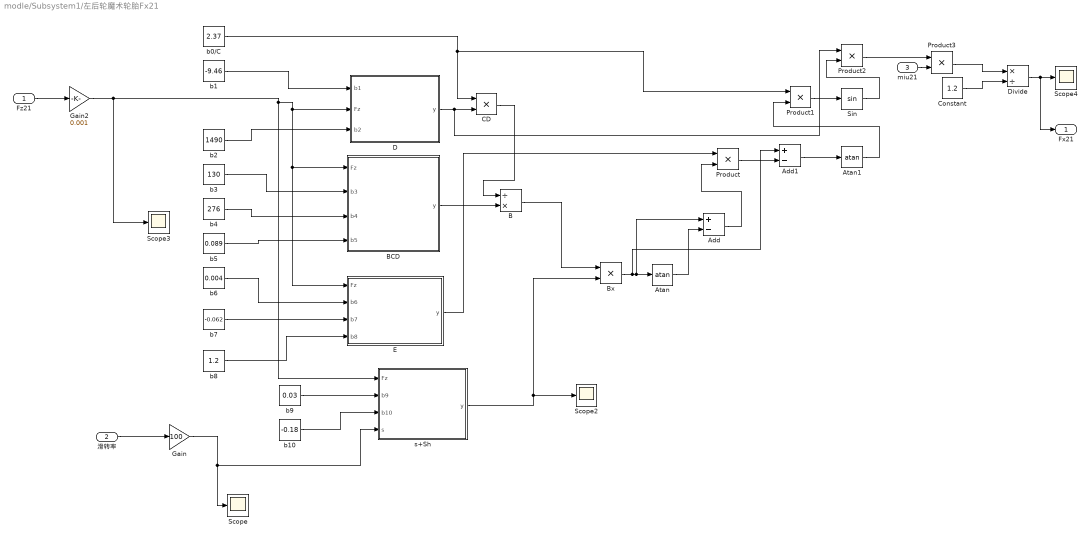
== system modle/Subsystem1/左后轮魔术轮胎Fx21 ==
  Fz21 : Inport
  滑转率 : Inport  Port=2
  miu21 : Inport  Port=3
  Add : Sum  Inputs=+-
  Add1 : Sum  Inputs=+-
  Atan : Trigonometry  Operator=atan
  Atan1 : Trigonometry  Operator=atan
  B : Product  Inputs=/*
  BCD : MATLAB Function  TreatAsAtomicUnit=on
  Bx : Product
  CD : Product
  Constant : Constant  Value=1.2  SampleTime=-1
  D : MATLAB Function  TreatAsAtomicUnit=on
  Divide : Product  Inputs=*/
  E : MATLAB Function  TreatAsAtomicUnit=on
  Gain : Gain  Gain=100
  Gain2 : Gain  Gain=0.001
  Product{,1..3} (4 alike) : Product
  Scope{,2..4} (4 alike) : Scope
  Sin : Trigonometry
  b0/C : Constant  Value=2.37
  b1 : Constant  Value=-9.46
  b10 : Constant  Value=-0.18
  b2 : Constant  Value=1490
  b3 : Constant  Value=130
  b4 : Constant  Value=276
  b5 : Constant  Value=0.089
  b6 : Constant  Value=0.004
  b7 : Constant  Value=-0.062
  b8 : Constant  Value=1.2
  b9 : Constant  Value=0.03
  s+Sh : MATLAB Function  TreatAsAtomicUnit=on
  Fx21 : Outport
  wires:
  Gain2/1 -> Scope3/1, s+Sh/1(Fz), E/1(Fz), BCD/1(Fz), D/2(Fz)
  b4/1 -> BCD/3(b4)
  Gain/1 -> s+Sh/4(s), Scope/1
  Product1/1 -> Sin/1
  滑转率/1 -> Gain/1
  b5/1 -> BCD/4(b5)
  Atan1/1 -> Product1/2
  Product/1 -> Add1/2
  D/1(y) -> Product2/1, CD/2
  b8/1 -> E/4(b8)
  Fz21/1 -> Gain2/1
  BCD/1(y) -> B/2
  B/1 -> Bx/1
  Add/1 -> Product/2
  b9/1 -> s+Sh/2(b9)
  Add1/1 -> Atan1/1
  b6/1 -> E/2(b6)
  b1/1 -> D/1(b1)
  Sin/1 -> Product2/2
  CD/1 -> B/1
  E/1(y) -> Product/1
  s+Sh/1(y) -> Scope2/1, Bx/2
  b10/1 -> s+Sh/3(b10)
  b2/1 -> D/3(b2)
  b7/1 -> E/3(b7)
  b3/1 -> BCD/2(b3)
  b0/C/1 -> Product1/1, CD/1
  Atan/1 -> Add/2
  Bx/1 -> Add1/1, Add/1, Atan/1
  Product3/1 -> Divide/1
  Divide/1 -> Fx21/1, Scope4/1
  miu21/1 -> Product3/2
  Product2/1 -> Product3/1
  Constant/1 -> Divide/2

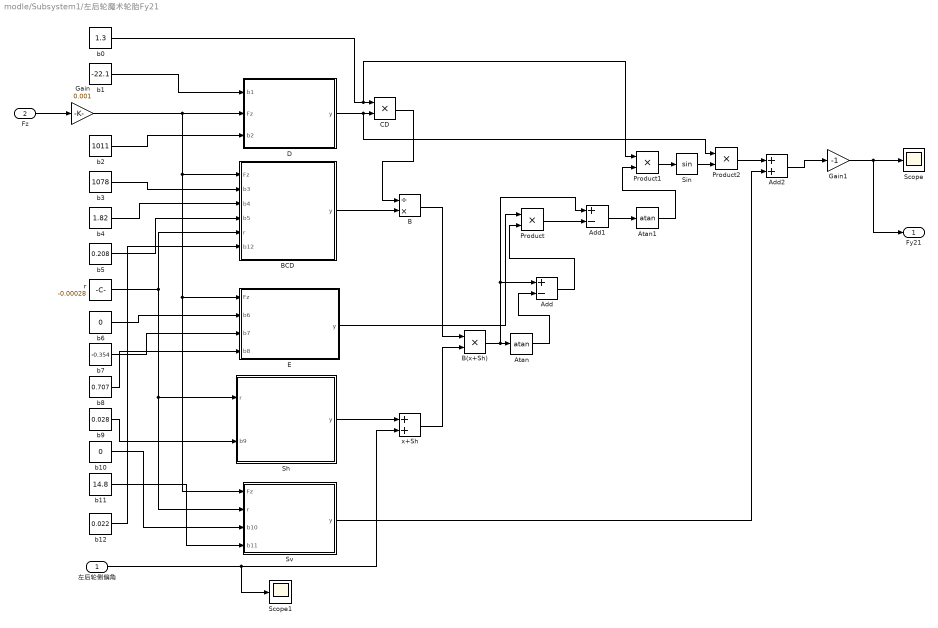
== system modle/Subsystem1/左后轮魔术轮胎Fy21 ==
  左后轮侧偏角 : Inport
  Fz : Inport  Port=2
  Add : Sum  Inputs=+-
  Add1 : Sum  Inputs=+-
  Add2 : Sum
  Atan : Trigonometry  Operator=atan
  Atan1 : Trigonometry  Operator=atan
  B : Product  Inputs=/*
  B(x+Sh) : Product
  BCD : MATLAB Function  TreatAsAtomicUnit=on
  CD : Product
  D : MATLAB Function  TreatAsAtomicUnit=on
  E : MATLAB Function  TreatAsAtomicUnit=on
  Gain : Gain  Gain=0.001
  Gain1 : Gain  Gain=-1
  Product : Product
  Product1 : Product
  Product2 : Product
  Scope : Scope
  Scope1 : Scope
  Sh : MATLAB Function  TreatAsAtomicUnit=on
  Sin : Trigonometry
  Sv : MATLAB Function  TreatAsAtomicUnit=on
  b0 : Constant  Value=1.3
  b1 : Constant  Value=-22.1
  b10 : Constant  Value=0
  b11 : Constant  Value=14.8
  b12 : Constant  Value=0.022
  b2 : Constant  Value=1011
  b3 : Constant  Value=1078
  b4 : Constant  Value=1.82
  b5 : Constant  Value=0.208
  b6 : Constant  Value=0
  b7 : Constant  Value=-0.354
  b8 : Constant  Value=0.707
  b9 : Constant  Value=0.028
  r : Constant  Value=-0.00028
  x+Sh : Sum
  Fy21 : Outport
  wires:
  Gain1/1 -> Fy21/1, Scope/1
  b9/1 -> Sh/2(b9)
  左后轮侧偏角/1 -> Scope1/1, x+Sh/2
  r/1 -> Sv/2(r), Sh/1(r), BCD/5(r)
  Fz/1 -> Gain/1
  Atan/1 -> Add/2
  b0/1 -> Product1/1, CD/1
  b12/1 -> BCD/6(b12)
  b8/1 -> E/4(b8)
  b11/1 -> Sv/4(b11)
  Sin/1 -> Product2/2
  b4/1 -> BCD/3(b4)
  Add/1 -> Product/2
  B(x+Sh)/1 -> Add/1, Add1/1, Atan/1
  Sh/1(y) -> x+Sh/1
  D/1(y) -> Product2/1, CD/2
  B/1 -> B(x+Sh)/1
  Atan1/1 -> Product1/2
  b7/1 -> E/3(b7)
  CD/1 -> B/1
  b6/1 -> E/2(b6)
  BCD/1(y) -> B/2
  x+Sh/1 -> B(x+Sh)/2
  Product1/1 -> Sin/1
  E/1(y) -> Product/1
  Product/1 -> Add1/2
  b5/1 -> BCD/4(b5)
  Add1/1 -> Atan1/1
  b3/1 -> BCD/2(b3)
  b2/1 -> D/3(b2)
  b1/1 -> D/1(b1)
  b10/1 -> Sv/3(b10)
  Product2/1 -> Add2/1
  Sv/1(y) -> Add2/2
  Add2/1 -> Gain1/1
  Gain/1 -> Sv/1(Fz), E/1(Fz), BCD/1(Fz), D/2(Fz)

== matlab function modle/Subsystem1/右后轮魔术轮胎Fx22/E ==
  data: Fz input; y output; b6 input; b7 input; b8 input
function y = fcn(Fz,b6,b7,b8)

y = b6*Fz*Fz+b7*Fz+b8;

== matlab function modle/Subsystem1/MATLAB Function7 ==
  data: X input; miu22 output
function miu22 = get_slope(X)
    % 根据车辆位置X计算道路坡度cta
    % 输入:
    %   X - 车辆位置（米）
    % 输出:
    %   cta - 道路坡度

    if X >= 0 && X <= 30
        miu22 = 0.3;
    elseif X > 30 && X <= 60
        miu22 = 0.3;
    elseif X > 60 && X <= 100
        miu22 = 0.3;
    else
        error('X is out of the defined range (0 - 200 meters)');
    end
end

== matlab function modle/Subsystem3/MATLAB Function ==
  data: x input; y output
function y = sgn(x)
    % sgn 返回输入 x 的符号
    % 如果 x > 0，则返回 1
    % 如果 x < 0，则返回 -1
    % 如果 x == 0，则返回 0
    
    y = zeros(size(x)); % 初始化输出变量
    y(x > 0) = 1;       % 对于 x > 0 的部分，设置 y 为 1
    y(x < 0) = -1;      % 对于 x < 0 的部分，设置 y 为 -1
    % 对于 x == 0 的部分，y 已经初始化为 0，无需额外设置
    
end

== matlab function modle/Subsystem1/MATLAB Function8 ==
  data: X input; miu21 output
function miu21 = get_slope(X)
    % 根据车辆位置X计算道路坡度cta
    % 输入:
    %   X - 车辆位置（米）
    % 输出:
    %   cta - 道路坡度

    if X >= 0 && X <= 30
        miu21 = 0.3;
    elseif X > 30 && X <= 60
        miu21 = 0.3;
    elseif X > 60 && X <= 100
        miu21 = 0.3;
    else
        error('X is out of the defined range (0 - 100 meters)');
    end
end

== matlab function modle/Subsystem1/右后轮魔术轮胎Fx22/s+Sh ==
  data: Fz input; b9 input; b10 input; s input; y output
function y = fcn(Fz,b9,b10,s)

y =s+b9*Fz+b10;

== matlab function modle/Subsystem1/左前轮魔术轮胎Fx11/BCD ==
  data: Fz input; y output; b3 input; b4 input; b5 input
function y = fcn(Fz,b3,b4,b5)

y = (b3*Fz*Fz+b4*Fz)*exp(-b5*Fz);

== matlab function modle/Subsystem1/MATLAB Function ==
  data: Fx11 input; ax output; Fx12 input; Fx21 input; Fx22 input; O11 input; O12 input; Fy11 input; Fy12 input; Fy21 input; Fy22 input; Fi input; Fw input; Ff input; Vx input; ay output; rdt output; Vy input; r input; m input; lf input; lr input; Bl input; Br input; Iz input; Fbu input
function [ax,ay,rdt] = fcn(Fx11,Fx12,Fx21,Fx22,O11,O12,Fy11,Fy12,Fy21,Fy22,Fi,Fw,Ff,Vx,Vy,r,m,lf,lr,Bl,Br,Iz,Fbu)
ax = (Fx11*cos(O11)+Fx12*cos(O12)-Fy11*sin(O11)-Fy12*sin(O12)+Fx21+Fx22-Fi-Fw-Ff+Fbu)/m+Vy*r;
ay = (Fx11*sin(O11)+Fx12*sin(O12)+Fy11*cos(O11)+Fy12*cos(O12)+Fy21+Fy22)/m-Vx*r;
rdt = (lf*(Fy11*cos(O11)+Fy12*cos(O12)+Fx11*sin(O11)+Fx12*sin(O12))-lr*(Fy21+Fy22)+Bl*(Fy11*sin(O11)-Fx11*cos(O11)-Fx21)+Br*(Fx12*cos(O12)-Fy12*sin(O12)+Fx22))/Iz;

== matlab function modle/Subsystem1/Fz11 ==
  data: lr input; Br input; m input; y output; g input; cta input; l input; B input; hg input; ax input; ay input
function y = fcn(lr,Br,m,g,cta,l,B,hg,ax,ay)

y = (lr*Br*m*g*cos(cta))/(l*B)-(lr*Br*m*g*hg*sin(cta))/(l*B)-(m*ax*hg)/(2*l)-(lr*m*ay*hg)/(l*B);

== matlab function modle/Subsystem1/Fz12 ==
  data: lr input; Bl input; m input; g input; cta input; y output; l input; B input; hg input; ax input; ay input
function y = fcn(lr,Bl,m,g,cta,l,B,hg,ax,ay)

y = (lr*Bl*m*g*cos(cta))/(l*B)-(lr*Bl*m*g*hg*sin(cta))/(l*B)-(m*ax*hg)/(2*l)+(lr*m*ay*hg)/(l*B);

== matlab function modle/Subsystem1/Fz21 ==
  data: lf input; Br input; m input; g input; cta input; y output; l input; B input; hg input; ax input; ay input
function y = fcn(lf,Br,m,g,cta,l,B,hg,ax,ay)

y = (lf*Br*m*g*cos(cta))/(l*B)+(lf*Br*m*g*hg*sin(cta))/(l*B)+(m*ax*hg)/(2*l)-(lf*m*ay*hg)/(l*B);

== matlab function modle/Subsystem1/左后轮魔术轮胎Fx21/BCD ==
  data: Fz input; y output; b3 input; b4 input; b5 input
function y = fcn(Fz,b3,b4,b5)

y = (b3*Fz*Fz+b4*Fz)*exp(-b5*Fz);

== matlab function modle/Subsystem1/左后轮魔术轮胎Fx21/D ==
  data: b1 input; y output; Fz input; b2 input
function y = fcn(b1,Fz,b2)

y = b1*Fz*Fz+b2*Fz+0.001;

== matlab function modle/Subsystem1/左后轮魔术轮胎Fx21/E ==
  data: Fz input; y output; b6 input; b7 input; b8 input
function y = fcn(Fz,b6,b7,b8)

y = b6*Fz*Fz+b7*Fz+b8;

== matlab function modle/Subsystem1/左后轮魔术轮胎Fx21/s+Sh ==
  data: Fz input; b9 input; b10 input; s input; y output
function y = fcn(Fz,b9,b10,s)

y =s+b9*Fz+b10;

== matlab function modle/MATLAB Function4 ==
  data: cta input; TM output; Vx input; am input
function  TM= fcn(cta,Vx,am)

TM =(1412*9.8*0*cos(cta)+0.25*2.2*Vx*Vx/21.15+1412*9.8*sin(cta)+1412*am)*0.325 ;

== matlab function modle/Subsystem1/MATLAB Function9 ==
  data: X input; miu11 output
function miu11 = get_slope(X)
    % 根据车辆位置X计算道路坡度cta
    % 输入:
    %   X - 车辆位置（米）
    % 输出:
    %   cta - 道路坡度

    if X >= 0 && X <= 30
        miu11 = 0.3;
    elseif X > 30 && X <= 60
        miu11 = 0.3;
    elseif X > 60 && X <= 100
        miu11 = 0.3;
    else
        error('X is out of the defined range (0 - 100 meters)');
    end
end

== matlab function modle/Subsystem1/MATLAB Function2 ==
  data: Fbu input; output output
function output = check_Fbu(Fbu)
    % check_Fbu - 检查Fbu值并输出结果
    % 输入参数:
    %   Fbu - 输入的Fbu值
    
    % 判断Fbu是否大于0
    if Fbu > 0
        output = Fbu;  % 符合条件，输出Fbu
    else
        output = 0;    % 不符合条件，输出0
    end
end

== matlab function modle/MATLAB Function6 ==
  data: X input; podu output
function podu = get_slope(X)
    % 根据车辆位置X计算道路坡度cta
    % 输入:
    %   X - 车辆位置（米）
    % 输出:
    %   cta - 道路坡度

    if X >= 0 && X <= 30
        podu = 0;
    elseif X > 30 && X <= 60
        podu = 0;
    elseif X > 60 && X <= 100
        podu = 0;
    else
        error('X is out of the defined range (0 - 100 meters)');
    end
end

== matlab function modle/MATLAB Function1 ==
  data: X input; miu12 output
function miu12 = get_slope(X)
    % 根据车辆位置X计算道路坡度cta
    % 输入:
    %   X - 车辆位置（米）
    % 输出:
    %   cta - 道路坡度

    if X >= 0 && X <= 30
        miu12 = 0.3;
    elseif X > 30 && X <= 60
        miu12 = 0.3;
    elseif X > 60 && X <= 100
        miu12 = 0.3;
    else
        error('X is out of the defined range (0 - 100 meters)');
    end
end

== matlab function modle/MATLAB Function7 ==
  data: X input; miu22 output
function miu22 = get_slope(X)
    % 根据车辆位置X计算道路坡度cta
    % 输入:
    %   X - 车辆位置（米）
    % 输出:
    %   cta - 道路坡度

    if X >= 0 && X <= 30
        miu22 = 0.3;
    elseif X > 30 && X <= 60
        miu22 = 0.3;
    elseif X > 60 && X <= 100
        miu22 = 0.3;
    else
        error('X is out of the defined range (0 - 200 meters)');
    end
end

== matlab function modle/Subsystem1/Fz22 ==
  data: lf input; Bl input; m input; g input; cta input; y output; l input; B input; hg input; ax input; ay input
function y = fcn(lf,Bl,m,g,cta,l,B,hg,ax,ay)

y = (lf*Bl*m*g*cos(cta))/(l*B)+(lf*Bl*m*g*hg*sin(cta))/(l*B)+(m*ax*hg)/(2*l)+(lf*m*ay*hg)/(l*B);

== matlab function modle/MATLAB Function8 ==
  data: X input; miu21 output
function miu21 = get_slope(X)
    % 根据车辆位置X计算道路坡度cta
    % 输入:
    %   X - 车辆位置（米）
    % 输出:
    %   cta - 道路坡度

    if X >= 0 && X <= 30
        miu21 = 0.3;
    elseif X > 30 && X <= 60
        miu21 = 0.3;
    elseif X > 60 && X <= 100
        miu21 = 0.3;
    else
        error('X is out of the defined range (0 - 100 meters)');
    end
end

== matlab function modle/MATLAB Function9 ==
  data: X input; miu11 output
function miu11 = get_slope(X)
    % 根据车辆位置X计算道路坡度cta
    % 输入:
    %   X - 车辆位置（米）
    % 输出:
    %   cta - 道路坡度

    if X >= 0 && X <= 30
        miu11 = 0.3;
    elseif X > 30 && X <= 60
        miu11 = 0.3;
    elseif X > 60 && X <= 100
        miu11 = 0.3;
    else
        error('X is out of the defined range (0 - 100 meters)');
    end
end

== matlab function modle/Subsystem1/前轮侧偏角 ==
  data: beta input; a input; Wr input; Vx input; u input; y output
function y = fcn(beta,a,Wr,Vx,u)

y = beta+a*Wr/Vx-u;

== matlab function modle/Subsystem1/前轮侧偏角1 ==
  data: beta input; a input; Wr input; Vx input; u input; y output
function y = fcn(beta,a,Wr,Vx,u)

y = beta+a*Wr/Vx-u;

== matlab function modle/Subsystem1/后轮侧偏角 ==
  data: beta input; b input; Wr input; Vx input; y output; u input
function y = fcn(beta,b,Wr,Vx,u)

y = beta-b*Wr/Vx+0.2*u;

== matlab function modle/Subsystem1/后轮侧偏角1 ==
  data: beta input; b input; Wr input; Vx input; y output; u input
function y = fcn(beta,b,Wr,Vx,u)

y = beta-b*Wr/Vx+0.2*u;

== matlab function modle/Subsystem3/MATLAB Function3 ==
  data: x input; y output
function y = sgn(x)
    % sgn 返回输入 x 的符号
    % 如果 x > 0，则返回 1
    % 如果 x < 0，则返回 -1
    % 如果 x == 0，则返回 0
    
    y = zeros(size(x)); % 初始化输出变量
    y(x > 0) = 1;       % 对于 x > 0 的部分，设置 y 为 1
    y(x < 0) = -1;      % 对于 x < 0 的部分，设置 y 为 -1
    % 对于 x == 0 的部分，y 已经初始化为 0，无需额外设置
    
end

== matlab function modle/Subsystem1/右前轮魔术轮胎Fy12/BCD ==
  data: Fz input; y output; b3 input; b4 input; b5 input; r input; b12 input
function y = fcn(Fz,b3,b4,b5,r,b12)

y = b3*sin(b4*atan(b5*Fz))*(1-b12*r);

== matlab function modle/Subsystem1/右前轮魔术轮胎Fy12/D ==
  data: b1 input; y output; Fz input; b2 input
function y = fcn(b1,Fz,b2)

y = b1*Fz*Fz+b2*Fz;

== matlab function modle/Subsystem1/右前轮魔术轮胎Fy12/E ==
  data: Fz input; y output; b6 input; b7 input; b8 input
function y = fcn(Fz,b6,b7,b8)

y = b6*Fz*Fz+b7*Fz+b8;

== matlab function modle/Subsystem1/右前轮魔术轮胎Fy12/Sh ==
  data: y output; r input; b9 input
function y = fcn(r,b9)

y = b9*r;

== matlab function modle/Subsystem1/右前轮魔术轮胎Fy12/Sv ==
  data: Fz input; y output; r input; b10 input; b11 input
function y = fcn(Fz,r,b10,b11)

y = (b10*Fz*Fz+b11*Fz)*r;

== matlab function modle/Subsystem1/右前轮魔术轮胎Fx12/BCD ==
  data: Fz input; y output; b3 input; b4 input; b5 input
function y = fcn(Fz,b3,b4,b5)

y = (b3*Fz*Fz+b4*Fz)*exp(-b5*Fz);

== matlab function modle/Subsystem1/右前轮魔术轮胎Fx12/D ==
  data: b1 input; y output; Fz input; b2 input
function y = fcn(b1,Fz,b2)

y = b1*Fz*Fz+b2*Fz+0.001;

== matlab function modle/Subsystem1/右后轮魔术轮胎Fy22/BCD ==
  data: Fz input; y output; b3 input; b4 input; b5 input; r input; b12 input
function y = fcn(Fz,b3,b4,b5,r,b12)

y = b3*sin(b4*atan(b5*Fz))*(1-b12*r);

== matlab function modle/Subsystem1/右后轮魔术轮胎Fy22/D ==
  data: b1 input; y output; Fz input; b2 input
function y = fcn(b1,Fz,b2)

y = b1*Fz*Fz+b2*Fz;

== matlab function modle/Subsystem1/右前轮魔术轮胎Fx12/E ==
  data: Fz input; y output; b6 input; b7 input; b8 input
function y = fcn(Fz,b6,b7,b8)

y = b6*Fz*Fz+b7*Fz+b8;

== matlab function modle/Subsystem1/右后轮魔术轮胎Fy22/E ==
  data: Fz input; y output; b6 input; b7 input; b8 input
function y = fcn(Fz,b6,b7,b8)

y = b6*Fz*Fz+b7*Fz+b8;

== matlab function modle/Subsystem1/右后轮魔术轮胎Fy22/Sh ==
  data: y output; r input; b9 input
function y = fcn(r,b9)

y = b9*r;

== matlab function modle/Subsystem1/右后轮魔术轮胎Fy22/Sv ==
  data: Fz input; y output; r input; b10 input; b11 input
function y = fcn(Fz,r,b10,b11)

y = (b10*Fz*Fz+b11*Fz)*r;

== matlab function modle/Subsystem1/左前轮魔术轮胎Fx11/D ==
  data: b1 input; y output; Fz input; b2 input
function y = fcn(b1,Fz,b2)

y = b1*Fz*Fz+b2*Fz+0.001;

== matlab function modle/Subsystem1/左前轮魔术轮胎Fx11/E ==
  data: Fz input; y output; b6 input; b7 input; b8 input
function y = fcn(Fz,b6,b7,b8)

y = b6*Fz*Fz+b7*Fz+b8;

== matlab function modle/Subsystem1/左前轮魔术轮胎Fx11/s+Sh ==
  data: Fz input; b9 input; b10 input; s input; y output
function y = fcn(Fz,b9,b10,s)

y =s+b9*Fz+b10;

== matlab function modle/Subsystem1/左前轮魔术轮胎Fy11/BCD ==
  data: Fz input; y output; b3 input; b4 input; b5 input; r input; b12 input
function y = fcn(Fz,b3,b4,b5,r,b12)

y = b3*sin(b4*atan(b5*Fz))*(1-b12*r);

== matlab function modle/Subsystem1/左前轮魔术轮胎Fy11/D ==
  data: b1 input; y output; Fz input; b2 input
function y = fcn(b1,Fz,b2)

y = b1*Fz*Fz+b2*Fz;

== matlab function modle/Subsystem1/左前轮魔术轮胎Fy11/E ==
  data: Fz input; y output; b6 input; b7 input; b8 input
function y = fcn(Fz,b6,b7,b8)

y = b6*Fz*Fz+b7*Fz+b8;

== matlab function modle/Subsystem1/左前轮魔术轮胎Fy11/Sh ==
  data: y output; r input; b9 input
function y = fcn(r,b9)

y = b9*r;

== matlab function modle/Subsystem1/左前轮魔术轮胎Fy11/Sv ==
  data: Fz input; y output; r input; b10 input; b11 input
function y = fcn(Fz,r,b10,b11)

y = (b10*Fz*Fz+b11*Fz)*r;

== matlab function modle/Subsystem1/右前轮魔术轮胎Fx12/s+Sh ==
  data: Fz input; b9 input; b10 input; s input; y output
function y = fcn(Fz,b9,b10,s)

y =s+b9*Fz+b10;

== matlab function modle/Subsystem1/左后轮魔术轮胎Fy21/BCD ==
  data: Fz input; y output; b3 input; b4 input; b5 input; r input; b12 input
function y = fcn(Fz,b3,b4,b5,r,b12)

y = b3*sin(b4*atan(b5*Fz))*(1-b12*r);

== matlab function modle/Subsystem1/左后轮魔术轮胎Fy21/D ==
  data: b1 input; y output; Fz input; b2 input
function y = fcn(b1,Fz,b2)

y = b1*Fz*Fz+b2*Fz;

== matlab function modle/Subsystem1/左后轮魔术轮胎Fy21/E ==
  data: Fz input; y output; b6 input; b7 input; b8 input
function y = fcn(Fz,b6,b7,b8)

y = b6*Fz*Fz+b7*Fz+b8;

== matlab function modle/Subsystem1/左后轮魔术轮胎Fy21/Sh ==
  data: y output; r input; b9 input
function y = fcn(r,b9)

y = b9*r;

== matlab function modle/Subsystem1/左后轮魔术轮胎Fy21/Sv ==
  data: Fz input; y output; r input; b10 input; b11 input
function y = fcn(Fz,r,b10,b11)

y = (b10*Fz*Fz+b11*Fz)*r;
